simulink model "Laba22"  (R2020a)
settings: Solver=VariableStepAuto  StartTime=0.0  StopTime=10.0  RelTol=1e-3
settings Model: Creator=LinkL  LastModifiedBy=LinkL

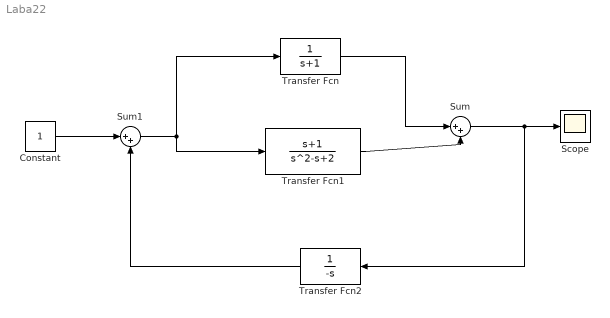
== system Laba22 ==
  Constant : Constant
  Scope : Scope
  Sum : Sum  Inputs=|++
  Sum1 : Sum  Inputs=|++
  Transfer Fcn : TransferFcn  Denominator=[1 1]
  Transfer Fcn1 : TransferFcn  Numerator=[1 1]  Denominator=[1 -1 2]
  Transfer Fcn2 : TransferFcn  Denominator=[-1 0]
  wires:
  Sum/1 -> Transfer Fcn2/1, Scope/1
  Transfer Fcn1/1 -> Sum/2
  Transfer Fcn/1 -> Sum/1
  Sum1/1 -> Transfer Fcn/1, Transfer Fcn1/1
  Constant/1 -> Sum1/1
  Transfer Fcn2/1 -> Sum1/2
